simulink model "ex_9_3"  (Simulink 10.1)
settings: Solver=ode23  StartTime=0.0  StopTime=3  FixedStep=0.001  RelTol=1e-3
values from neighbouring files (symbols this model uses):
  a1 = I1 + m1 * Icl^2 + Ie + me * Ice^2 + me * L1^2    (= 3.34)    [ex_9_1.m]    (also in ex_9_2.m; ex_9_3.m)
  a2 = Ie + me * Ice^2    (= 0.97)    [ex_9_1.m]    (also in ex_9_2.m; ex_9_3.m)
  a3 = me * L1 * Ice * cos(delta_e)    [ex_9_1.m]    (also in ex_9_2.m = me_hat * L1 * Ice * cos(delta_e); ex_9_3.m = me_hat * L1 * Ice * cos(delta_e))
  a4 = me * L1 * Ice * sin(delta_e)    [ex_9_1.m]    (also in ex_9_2.m = me_hat * L1 * Ice * sin(delta_e); ex_9_3.m = me_hat * L1 * Ice * sin(delta_e))
  delta_e = 30    [ex_9_1.m]    (also in ex_9_2.m = 0.523599; ex_9_3.m = 0.523599)
  I1 = 0.12    [ex_9_1.m]    (also in ex_9_2.m; ex_9_3.m)
  Ice = 0.6    [ex_9_1.m]    (also in ex_9_2.m; ex_9_3.m)
  Icl = 0.5    [ex_9_1.m]    (also in ex_9_2.m; ex_9_3.m)
  Ie = 0.25    [ex_9_1.m]    (also in ex_9_2.m; ex_9_3.m)
  L1 = 1    [ex_9_1.m]    (also in ex_9_2.m; ex_9_3.m)
libraries: dspmtrx3 x4
settings Model: Creator=Paulo Padrao  LastModifiedBy=Paulo Padrao
settings DataIOCC: SaveFormat=Dataset
settings OptimizationCC: LifeSpan=auto
settings DebuggingCC: UnderspecifiedInitializationDetection=Simplified  MergeDetectMultiDrivingBlocksExec=error  SFUnexpectedBacktrackingDiag=error  SFNoUnconditionalDefaultTransitionDiag=error  SFExecutionAtInitializationDiag=warning
settings HardwareCC: ProdBitPerPointer=64  ProdBitPerSizeT=64  ProdBitPerPtrDiffT=64  ProdLargestAtomicFloat=Float  ProdIntDivRoundTo=Zero  ProdEndianess=LittleEndian  ProdWordSize=64  ProdHWDeviceType=Intel->x86-64 (Windows64)
settings ModelReferenceCC: PropagateSignalLabelsOutOfModel=on
settings CodeAppCC: StateflowObjectComments=off
settings GRTTargetCC: TargetLangStandard=C99 (ISO)  CombineOutputUpdateFcns=on  GRTInterface=off
settings ConfigComp: CovMetricSettings=dwe  CovHtmlReporting=off  CovSaveCumulativeToWorkspaceVar=off  CovSaveSingleToWorkspaceVar=off  CovExternalEMLEnable=on

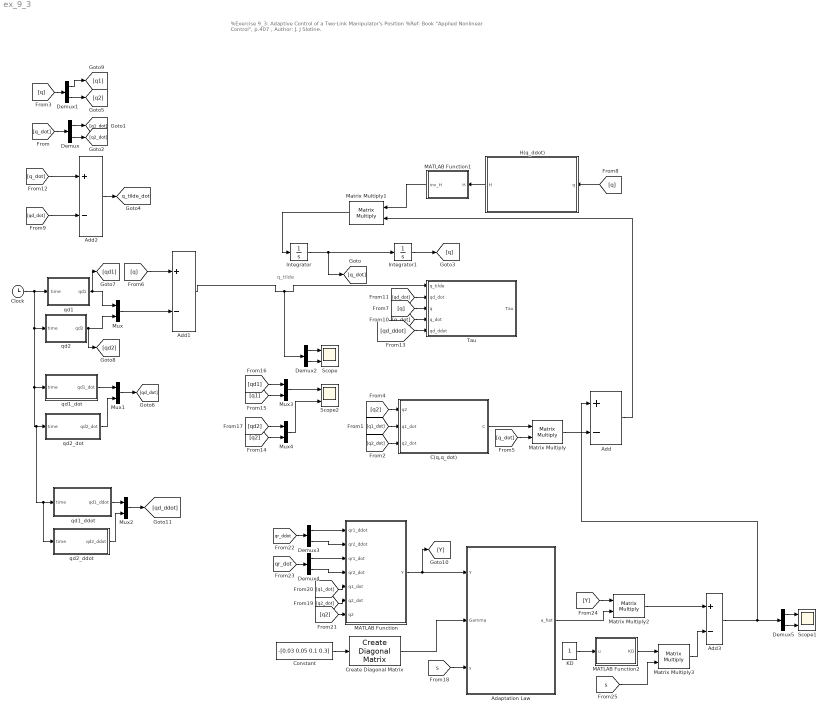
== system ex_9_3 ==
  note: %Exercise 9_3: Adaptive Control of a Two-Link Manipulator's Position
      | %Ref: Book "Applied Nonlinear Control", p.407 , Author: J. J Slotine.
  note: q_tilde
  Adaptation Law : Subsystem
  Add{,1..3} (4 alike) : Sum  Inputs=+-
  C(q,q_dot) : Subsystem
  Clock : Clock
  Constant : Constant  Value=-[0.03 0.05 0.1 0.3]
  Create Diagonal Matrix : dspmtrx3/Create Diagonal Matrix
      settings: SourceProductBaseCode=DS
  Demux{,1..5} (6 alike) : Demux  Outputs=2
  H(q_ddot) : Subsystem
  Integrator : Integrator
  Integrator1 : Integrator
  KD : Constant
  MATLAB Function : MATLAB Function  TreatAsAtomicUnit=on
  MATLAB Function1 : MATLAB Function  TreatAsAtomicUnit=on
  MATLAB Function2 : MATLAB Function  TreatAsAtomicUnit=on
  Matrix Multiply{,1..3} (4 alike) : Product  Multiplication=Matrix(*)
  Mux{,1..4} (5 alike) : Mux  Inputs=2
  Scope : Scope  NumInputPorts=2
  Scope1 : Scope  NumInputPorts=2
  Scope2 : Scope  NumInputPorts=2
  Tau : Subsystem
  qd1 : MATLAB Function  TreatAsAtomicUnit=on
  qd1_ddot : MATLAB Function  TreatAsAtomicUnit=on
  qd1_dot : MATLAB Function  TreatAsAtomicUnit=on
  qd2 : MATLAB Function  TreatAsAtomicUnit=on
  qd2_ddot : MATLAB Function  TreatAsAtomicUnit=on
  qd2_dot : MATLAB Function  TreatAsAtomicUnit=on
  tag scope: q_tilde_dot=global
  wires:
  Integrator/1 -> [q_dot], Integrator1/1
  [q_dot] -> Demux/1
  Demux/1 -> [q1_dot]
  Demux/2 -> [q2_dot]
  [q1_dot] -> C(q,q_dot)/2(q1_dot)
  [q2_dot] -> C(q,q_dot)/3(q2_dot)
  Integrator1/1 -> [q]
  [q] -> Demux1/1
  Demux1/2 -> [q2]
  [q2] -> C(q,q_dot)/1(q2)
  C(q,q_dot)/1(C) -> Matrix Multiply/1
  [q_dot] -> Matrix Multiply/2
  [q] -> H(q_ddot)/1(q)
  qd2/1(qd2) -> Mux/2, [qd2]
  [q] -> Add1/1
  Mux/1 -> Add1/2
  Add1/1 -> Demux2/1, Tau/1(q_tilde)
  [qd_dot] -> Tau/2(qd_dot)
  Demux1/1 -> [q1]
  Matrix Multiply/1 -> Add/2
  Matrix Multiply1/1 -> Integrator/1
  Add/1 -> Matrix Multiply1/2
  Demux2/2 -> Scope/2
  Demux2/1 -> Scope/1
  [q] -> Tau/3(q)
  [q_dot] -> Tau/4(q_dot)
  qd1_dot/1(qd1_dot) -> Mux1/1
  qd2_dot/1(qd2_dot) -> Mux1/2
  Mux1/1 -> [qd_dot]
  H(q_ddot)/1(H) -> MATLAB Function1/1(H)
  MATLAB Function1/1(inv_H) -> Matrix Multiply1/1
  [qd_dot] -> Add2/2
  [q_dot] -> Add2/1
  Add2/1 -> [q_tilde_dot]
  Clock/1 -> qd2_ddot/1(time), qd1_ddot/1(time), qd2_dot/1(time), qd1_dot/1(time), qd2/1(time), qd1/1(time)
  qd2_ddot/1(qd2_ddot) -> Mux2/2
  Mux2/1 -> [qd_ddot]
  qd1_ddot/1(qd1_ddot) -> Mux2/1
  [qd_ddot] -> Tau/5(qd_ddot)
  Mux3/1 -> Scope2/1
  qd1/1(qd1) -> Mux/1, [qd1]
  Mux4/1 -> Scope2/2
  [q2] -> Mux4/2
  [q1] -> Mux3/2
  [qd1] -> Mux3/1
  [qd2] -> Mux4/1
  Constant/1 -> Create Diagonal Matrix/1
  Create Diagonal Matrix/1 -> Adaptation Law/2(Gamma)
  [s] -> Adaptation Law/3(s)
  MATLAB Function/1(Y) -> [Y], Adaptation Law/1(Y)
  [q2_dot] -> MATLAB Function/6(q2_dot)
  [q1_dot] -> MATLAB Function/5(q1_dot)
  [q2] -> MATLAB Function/7(q2)
  [qr_ddot] -> Demux3/1
  Demux3/1 -> MATLAB Function/1(qr1_ddot)
  Demux3/2 -> MATLAB Function/2(qr2_ddot)
  Demux4/2 -> MATLAB Function/4(qr2_dot)
  Demux4/1 -> MATLAB Function/3(qr1_dot)
  [qr_dot] -> Demux4/1
  [Y] -> Matrix Multiply2/1
  Adaptation Law/1(a_hat) -> Matrix Multiply2/2
  Matrix Multiply2/1 -> Add3/1
  Demux5/1 -> Scope1/1
  Demux5/2 -> Scope1/2
  Add3/1 -> Add/1, Demux5/1
  Matrix Multiply3/1 -> Add3/2
  MATLAB Function2/1(KD) -> Matrix Multiply3/1
  [s] -> Matrix Multiply3/2
  KD/1 -> MATLAB Function2/1(u)

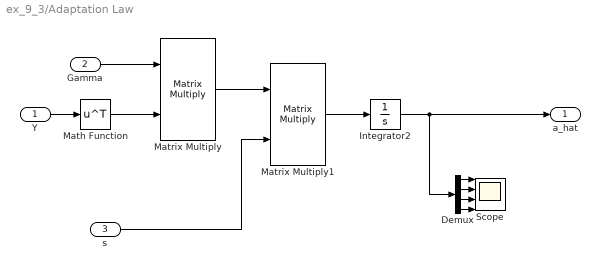
== system ex_9_3/Adaptation Law ==
  Y : Inport
  Gamma : Inport  Port=2
  s : Inport  Port=3
  Demux : Demux
  Integrator2 : Integrator
  Math Function : Math  Operator=transpose  SignedPower=on  SaturateOnIntegerOverflow=on
  Matrix Multiply : Product  Multiplication=Matrix(*)
  Matrix Multiply1 : Product  Multiplication=Matrix(*)
  Scope : Scope  NumInputPorts=4
  a_hat : Outport  VectorParamsAs1DForOutWhenUnconnected=off
  wires:
  Integrator2/1 -> Demux/1, a_hat/1
  Gamma/1 -> Matrix Multiply/1
  Math Function/1 -> Matrix Multiply/2
  Y/1 -> Math Function/1
  Matrix Multiply/1 -> Matrix Multiply1/1
  s/1 -> Matrix Multiply1/2
  Matrix Multiply1/1 -> Integrator2/1
  Demux/1 -> Scope/1
  Demux/2 -> Scope/2
  Demux/3 -> Scope/3
  Demux/4 -> Scope/4

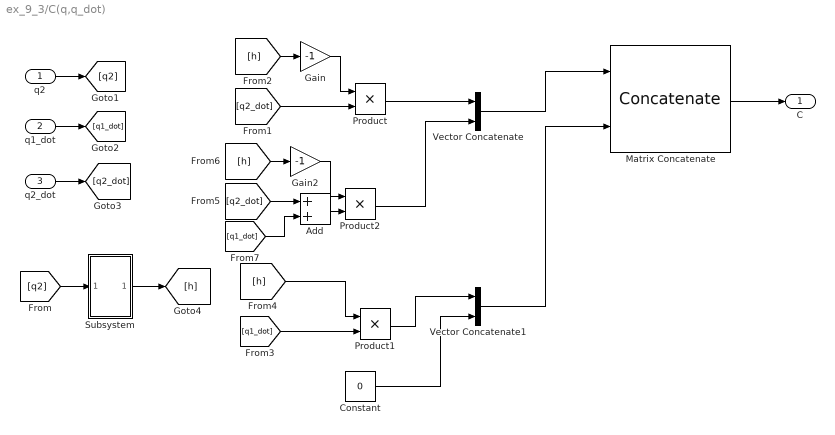
== system ex_9_3/C(q,q_dot) ==
  q2 : Inport
  q1_dot : Inport  Port=2
  q2_dot : Inport  Port=3
  Add : Sum
  Constant : Constant  Value=0
  Gain : Gain  Gain=-1
  Gain2 : Gain  Gain=-1
  Matrix Concatenate : Concatenate  Mode=Multidimensional array
  Product : Product
  Product1 : Product
  Product2 : Product
  Subsystem : Subsystem
  Vector Concatenate : Concatenate  Mode=Multidimensional array  ConcatenateDimension=2
  Vector Concatenate1 : Concatenate  Mode=Multidimensional array  ConcatenateDimension=2
  C : Outport  VectorParamsAs1DForOutWhenUnconnected=off
  wires:
  q2/1 -> [q2]
  q1_dot/1 -> [q1_dot]
  q2_dot/1 -> [q2_dot]
  [q2] -> Subsystem/1(In1)
  Subsystem/1(Out1) -> [h]
  Matrix Concatenate/1 -> C/1
  [q2_dot] -> Product/2
  [h] -> Gain/1
  Gain/1 -> Product/1
  [h] -> Product1/1
  [q1_dot] -> Product1/2
  Gain2/1 -> Product2/1
  [h] -> Gain2/1
  [q2_dot] -> Add/1
  [q1_dot] -> Add/2
  Add/1 -> Product2/2
  Product/1 -> Vector Concatenate/1
  Vector Concatenate/1 -> Matrix Concatenate/1
  Constant/1 -> Vector Concatenate1/2
  Vector Concatenate1/1 -> Matrix Concatenate/2
  Product2/1 -> Vector Concatenate/2
  Product1/1 -> Vector Concatenate1/1

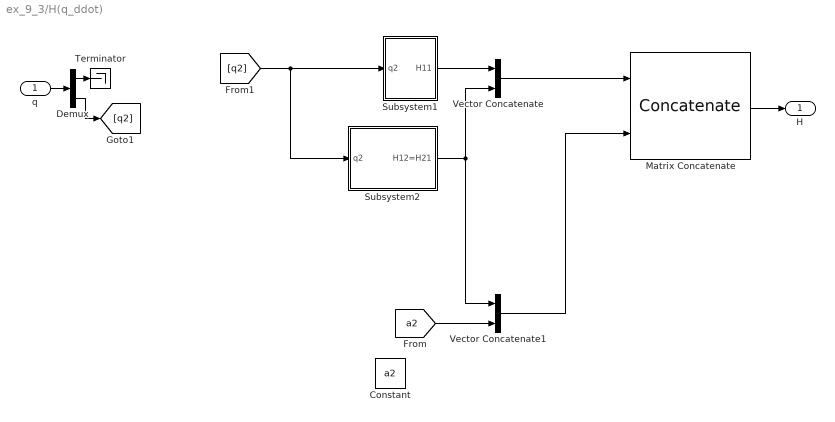
== system ex_9_3/H(q_ddot) ==
  q : Inport
  Constant : Constant  Value=a2
  Demux : Demux  Outputs=2
  Matrix Concatenate : Concatenate  Mode=Multidimensional array
  Subsystem1 : Subsystem
  Subsystem2 : Subsystem
  Terminator : Terminator
  Vector Concatenate : Concatenate  Mode=Multidimensional array  ConcatenateDimension=2
  Vector Concatenate1 : Concatenate  Mode=Multidimensional array  ConcatenateDimension=2
  H : Outport  VectorParamsAs1DForOutWhenUnconnected=off
  wires:
  q/1 -> Demux/1
  Demux/2 -> [q2]
  [q2] -> Subsystem1/1(q2), Subsystem2/1(q2)
  Subsystem2/1("H12=H21 ") -> Vector Concatenate1/1, Vector Concatenate/2
  Vector Concatenate1/1 -> Matrix Concatenate/2
  Subsystem1/1("H11 ") -> Vector Concatenate/1
  Vector Concatenate/1 -> Matrix Concatenate/1
  Demux/1 -> Terminator/1
  Matrix Concatenate/1 -> H/1
  [a2] -> Vector Concatenate1/2

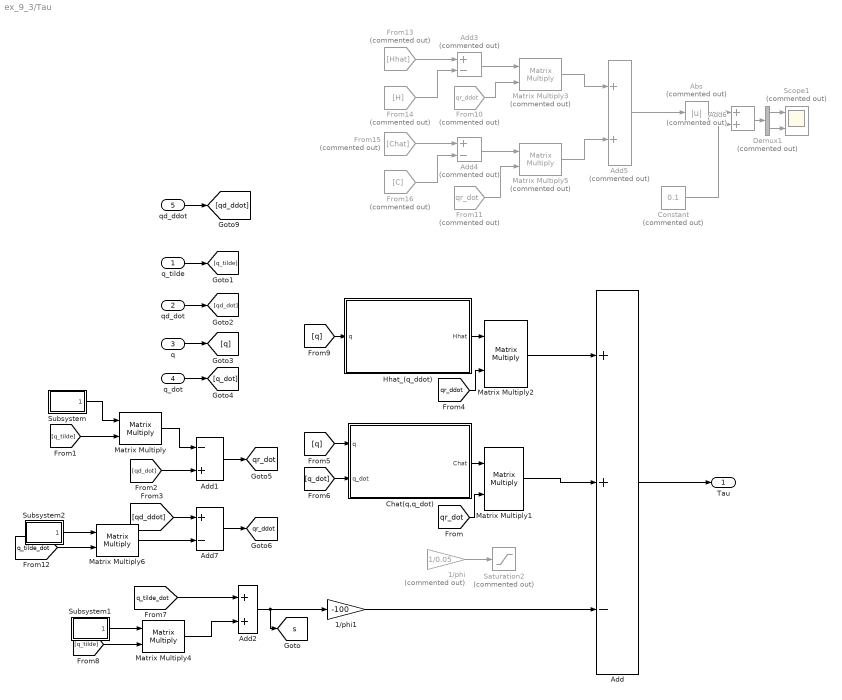
== system ex_9_3/Tau ==
  q_tilde : Inport
  qd_dot : Inport  Port=2
  q : Inport  Port=3
  q_dot : Inport  Port=4
  qd_ddot : Inport  Port=5
  1/phi : Gain  Commented=on  Gain=1/0.05
  1/phi1 : Gain  Gain=-100
  Abs : Abs  Commented=on  ZeroCross=off
  Add : Sum  Inputs=++-
  Add1 : Sum  Inputs=-+
  Add2 : Sum
  Add3 : Sum  Commented=on  Inputs=+-
  Add4 : Sum  Commented=on  Inputs=+-
  Add5 : Sum  Commented=on
  Add6 : Sum  Commented=on
  Add7 : Sum  Inputs=+-
  Chat(q,q_dot) : Subsystem
  Constant : Constant  Commented=on  Value=0.1
  Demux1 : Demux  Commented=on  Outputs=2
  From10 : From  Commented=on  GotoTag=qr_ddot
  From11 : From  Commented=on  GotoTag=qr_dot
  From13 : From  Commented=on  GotoTag=Hhat  TagVisibility=global
  From14 : From  Commented=on  GotoTag=H  TagVisibility=global
  From15 : From  Commented=on  GotoTag=Chat  TagVisibility=global
  From16 : From  Commented=on  GotoTag=C  TagVisibility=global
  Hhat_(q_ddot) : Subsystem
  Matrix Multiply{,1..2,4,6} (5 alike) : Product  Multiplication=Matrix(*)
  Matrix Multiply3 : Product  Commented=on  Multiplication=Matrix(*)
  Matrix Multiply5 : Product  Commented=on  Multiplication=Matrix(*)
  Saturation2 : Saturate  Commented=on  UpperLimit=0.1  LowerLimit=-0.1  LinearizeAsGain=off  ZeroCross=off
  Scope1 : Scope  Commented=on  NumInputPorts=2
  Subsystem : Subsystem
  Subsystem1 : Subsystem
  Subsystem2 : Subsystem
  Tau : Outport  VectorParamsAs1DForOutWhenUnconnected=off
  tag scope: qr_ddot=global, qr_dot=global, s=global
  wires:
  Add/1 -> Tau/1
  q_tilde/1 -> [q_tilde]
  qd_dot/1 -> [qd_dot]
  [q_tilde] -> Matrix Multiply/2
  q/1 -> [q]
  q_dot/1 -> [q_dot]
  Subsystem/1(lambda) -> Matrix Multiply/1
  Matrix Multiply/1 -> Add1/1
  Add1/1 -> [qr_dot]
  Matrix Multiply2/1 -> Add/1
  Matrix Multiply1/1 -> Add/2
  [qr_dot] -> Matrix Multiply1/2
  [qr_ddot] -> Matrix Multiply2/2
  Chat(q,q_dot)/1(Chat) -> Matrix Multiply1/1
  [q] -> Chat(q,q_dot)/1(q)
  [q_dot] -> Chat(q,q_dot)/2(q_dot)
  [q_tilde_dot] -> Add2/1
  Matrix Multiply4/1 -> Add2/2
  Hhat_(q_ddot)/1(Hhat) -> Matrix Multiply2/1
  [q] -> Hhat_(q_ddot)/1(q)
  [qd_dot] -> Add1/2
  Subsystem1/1(lambda) -> Matrix Multiply4/1
  [q_tilde] -> Matrix Multiply4/2
  1/phi/1 -> Saturation2/1
  From13/1 -> Add3/1
  From16/1 -> Add4/2
  From15/1 -> Add4/1
  Add3/1 -> Matrix Multiply3/1
  From14/1 -> Add3/2
  From10/1 -> Matrix Multiply3/2
  Add4/1 -> Matrix Multiply5/1
  From11/1 -> Matrix Multiply5/2
  Matrix Multiply3/1 -> Add5/1
  Matrix Multiply5/1 -> Add5/2
  Add5/1 -> Abs/1
  Abs/1 -> Add6/1
  Constant/1 -> Add6/2
  qd_ddot/1 -> [qd_ddot]
  Add7/1 -> [qr_ddot]
  [qd_ddot] -> Add7/1
  Matrix Multiply6/1 -> Add7/2
  Subsystem2/1(lambda) -> Matrix Multiply6/1
  [q_tilde_dot] -> Matrix Multiply6/2
  Add6/1 -> Demux1/1
  Demux1/1 -> Scope1/1
  Demux1/2 -> Scope1/2
  1/phi1/1 -> Add/3
  Add2/1 -> [s], 1/phi1/1

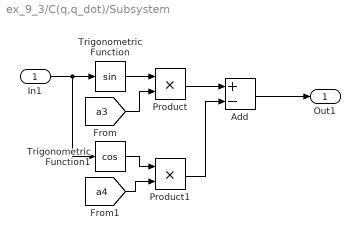
== system ex_9_3/C(q,q_dot)/Subsystem ==
  In1 : Inport
  Add : Sum  Inputs=+-
  Product : Product
  Product1 : Product
  Trigonometric Function : Trigonometry
  Trigonometric Function1 : Trigonometry  Operator=cos
  Out1 : Outport  VectorParamsAs1DForOutWhenUnconnected=off
  wires:
  Trigonometric Function1/1 -> Product1/1
  [a3] -> Product/2
  Product/1 -> Add/1
  [a4] -> Product1/2
  In1/1 -> Trigonometric Function1/1, Trigonometric Function/1
  Trigonometric Function/1 -> Product/1
  Add/1 -> Out1/1
  Product1/1 -> Add/2

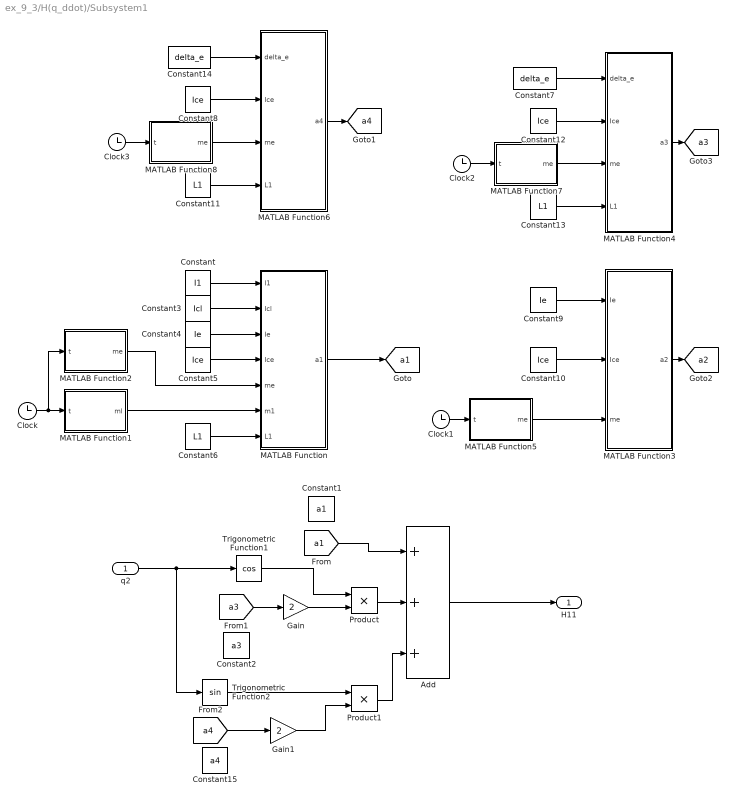
== system ex_9_3/H(q_ddot)/Subsystem1 ==
  q2 : Inport
  Add : Sum  Inputs=+++
  Clock{,1..3} (4 alike) : Clock
  Constant : Constant  Value=I1
  Constant1 : Constant  Value=a1
  Constant{5,8,10,12} (4 alike) : Constant  Value=Ice
  Constant11 : Constant  Value=L1
  Constant13 : Constant  Value=L1
  Constant14 : Constant  Value=delta_e
  Constant15 : Constant  Value=a4
  Constant2 : Constant  Value=a3
  Constant3 : Constant  Value=Icl
  Constant4 : Constant  Value=Ie
  Constant6 : Constant  Value=L1
  Constant7 : Constant  Value=delta_e
  Constant9 : Constant  Value=Ie
  Gain : Gain  Gain=2
  Gain1 : Gain  Gain=2
  MATLAB Function : MATLAB Function  TreatAsAtomicUnit=on
  MATLAB Function1 : MATLAB Function  TreatAsAtomicUnit=on
  MATLAB Function2 : MATLAB Function  TreatAsAtomicUnit=on
  MATLAB Function3 : MATLAB Function  TreatAsAtomicUnit=on
  MATLAB Function4 : MATLAB Function  TreatAsAtomicUnit=on
  MATLAB Function5 : MATLAB Function  TreatAsAtomicUnit=on
  MATLAB Function6 : MATLAB Function  TreatAsAtomicUnit=on
  MATLAB Function7 : MATLAB Function  TreatAsAtomicUnit=on
  MATLAB Function8 : MATLAB Function  TreatAsAtomicUnit=on
  Product : Product
  Product1 : Product
  Trigonometric Function1 : Trigonometry  Operator=cos
  Trigonometric Function2 : Trigonometry
  "H11 " : Outport  VectorParamsAs1DForOutWhenUnconnected=off
  tag scope: a1=global, a2=global, a3=global, a4=global
  wires:
  q2/1 -> Trigonometric Function1/1, Trigonometric Function2/1
  Add/1 -> "H11 "/1
  Product/1 -> Add/2
  Trigonometric Function1/1 -> Product/1
  Trigonometric Function2/1 -> Product1/1
  Product1/1 -> Add/3
  Constant/1 -> MATLAB Function/1(I1)
  Constant3/1 -> MATLAB Function/2(Icl)
  Constant4/1 -> MATLAB Function/3(Ie)
  Constant5/1 -> MATLAB Function/4(Ice)
  Constant6/1 -> MATLAB Function/7(L1)
  Clock/1 -> MATLAB Function2/1(t), MATLAB Function1/1(t)
  MATLAB Function1/1(ml) -> MATLAB Function/6(m1)
  MATLAB Function2/1(me) -> MATLAB Function/5(me)
  MATLAB Function5/1(me) -> MATLAB Function3/3(me)
  Clock1/1 -> MATLAB Function5/1(t)
  Constant10/1 -> MATLAB Function3/2(Ice)
  Constant9/1 -> MATLAB Function3/1(Ie)
  MATLAB Function7/1(me) -> MATLAB Function4/3(me)
  Clock2/1 -> MATLAB Function7/1(t)
  Constant13/1 -> MATLAB Function4/4(L1)
  Constant12/1 -> MATLAB Function4/2(Ice)
  Constant7/1 -> MATLAB Function4/1(delta_e)
  Constant14/1 -> MATLAB Function6/1(delta_e)
  Constant8/1 -> MATLAB Function6/2(Ice)
  Constant11/1 -> MATLAB Function6/4(L1)
  Clock3/1 -> MATLAB Function8/1(t)
  MATLAB Function8/1(me) -> MATLAB Function6/3(me)
  MATLAB Function/1(a1) -> [a1]
  MATLAB Function6/1(a4) -> [a4]
  MATLAB Function3/1(a2) -> [a2]
  MATLAB Function4/1(a3) -> [a3]
  Gain/1 -> Product/2
  Gain1/1 -> Product1/2
  [a4] -> Gain1/1
  [a3] -> Gain/1
  [a1] -> Add/1

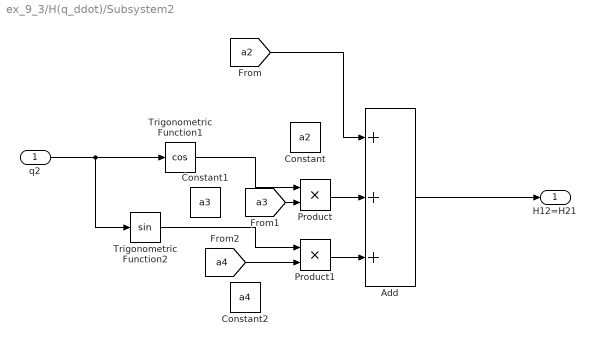
== system ex_9_3/H(q_ddot)/Subsystem2 ==
  q2 : Inport
  Add : Sum  Inputs=+++
  Constant : Constant  Value=a2
  Constant1 : Constant  Value=a3
  Constant2 : Constant  Value=a4
  Product : Product
  Product1 : Product
  Trigonometric Function1 : Trigonometry  Operator=cos
  Trigonometric Function2 : Trigonometry
  "H12=H21 " : Outport  VectorParamsAs1DForOutWhenUnconnected=off
  wires:
  Product1/1 -> Add/3
  Trigonometric Function2/1 -> Product1/1
  Trigonometric Function1/1 -> Product/1
  Product/1 -> Add/2
  Add/1 -> "H12=H21 "/1
  q2/1 -> Trigonometric Function2/1, Trigonometric Function1/1
  [a4] -> Product1/2
  [a3] -> Product/2
  [a2] -> Add/1

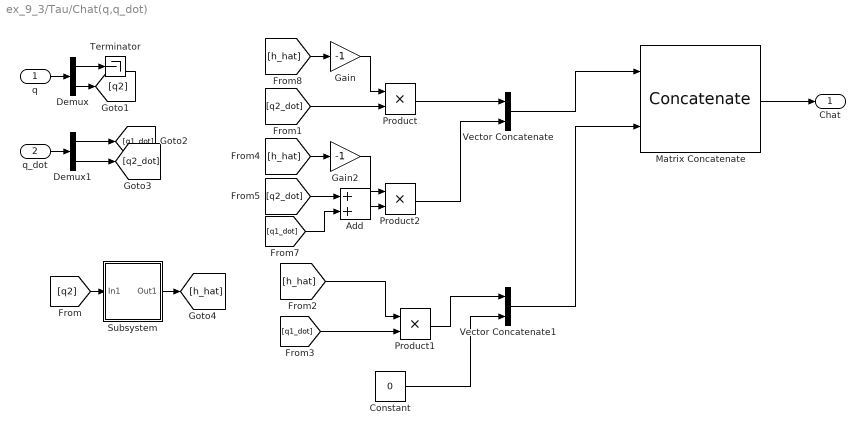
== system ex_9_3/Tau/Chat(q,q_dot) ==
  q : Inport
  q_dot : Inport  Port=2
  Add : Sum
  Constant : Constant  Value=0
  Demux : Demux  Outputs=2
  Demux1 : Demux  Outputs=2
  Gain : Gain  Gain=-1
  Gain2 : Gain  Gain=-1
  Matrix Concatenate : Concatenate  Mode=Multidimensional array
  Product : Product
  Product1 : Product
  Product2 : Product
  Subsystem : Subsystem
  Terminator : Terminator
  Vector Concatenate : Concatenate  Mode=Multidimensional array  ConcatenateDimension=2
  Vector Concatenate1 : Concatenate  Mode=Multidimensional array  ConcatenateDimension=2
  Chat : Outport  VectorParamsAs1DForOutWhenUnconnected=off
  wires:
  [q2] -> Subsystem/1(In1)
  Subsystem/1(Out1) -> [h_hat]
  Matrix Concatenate/1 -> Chat/1
  [q2_dot] -> Product/2
  [h_hat] -> Gain/1
  Gain/1 -> Product/1
  [h_hat] -> Product1/1
  [q1_dot] -> Product1/2
  Gain2/1 -> Product2/1
  [h_hat] -> Gain2/1
  [q2_dot] -> Add/1
  [q1_dot] -> Add/2
  Add/1 -> Product2/2
  Product/1 -> Vector Concatenate/1
  Vector Concatenate/1 -> Matrix Concatenate/1
  Constant/1 -> Vector Concatenate1/2
  Vector Concatenate1/1 -> Matrix Concatenate/2
  q/1 -> Demux/1
  Demux/2 -> [q2]
  Demux/1 -> Terminator/1
  q_dot/1 -> Demux1/1
  Demux1/2 -> [q2_dot]
  Demux1/1 -> [q1_dot]
  Product1/1 -> Vector Concatenate1/1
  Product2/1 -> Vector Concatenate/2

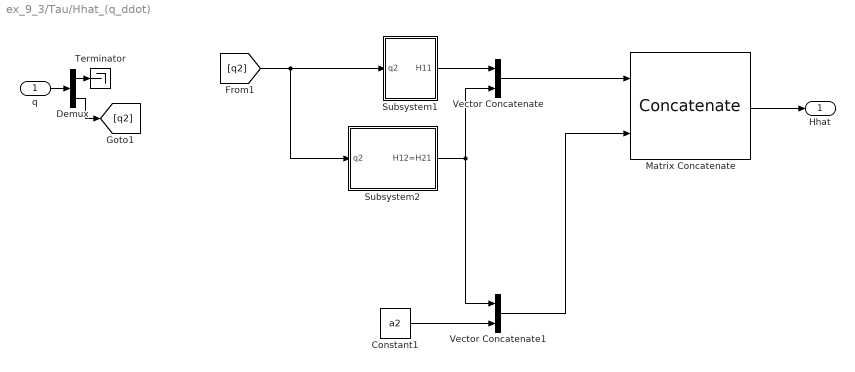
== system ex_9_3/Tau/Hhat_(q_ddot) ==
  q : Inport
  Constant1 : Constant  Value=a2
  Demux : Demux  Outputs=2
  Matrix Concatenate : Concatenate  Mode=Multidimensional array
  Subsystem1 : Subsystem
  Subsystem2 : Subsystem
  Terminator : Terminator
  Vector Concatenate : Concatenate  Mode=Multidimensional array  ConcatenateDimension=2
  Vector Concatenate1 : Concatenate  Mode=Multidimensional array  ConcatenateDimension=2
  Hhat : Outport  VectorParamsAs1DForOutWhenUnconnected=off
  wires:
  Vector Concatenate1/1 -> Matrix Concatenate/2
  Vector Concatenate/1 -> Matrix Concatenate/1
  Matrix Concatenate/1 -> Hhat/1
  Subsystem1/1("H11 ") -> Vector Concatenate/1
  [q2] -> Subsystem1/1(q2), Subsystem2/1(q2)
  Constant1/1 -> Vector Concatenate1/2
  Subsystem2/1("H12=H21 ") -> Vector Concatenate1/1, Vector Concatenate/2
  q/1 -> Demux/1
  Demux/2 -> [q2]
  Demux/1 -> Terminator/1

== system ex_9_3/Tau/Subsystem ==
  Identity Matrix2 : dspmtrx3/Identity Matrix  Inherit=off  N=2  Ts=1  dataType=double  isSigned=on  wordLen=16  udDataType=sfix(16)  fracBitsMode=Best precision  numFracBits=15  OutDataTypeStr=double  LastOutDataTypeStr=double
  LAMBDA : Constant  Value=20
  Product1 : Product
  lambda : Outport  VectorParamsAs1DForOutWhenUnconnected=off
  wires:
  Identity Matrix2/1 -> Product1/1
  LAMBDA/1 -> Product1/2
  Product1/1 -> lambda/1

== system ex_9_3/Tau/Subsystem1 ==
  Identity Matrix2 : dspmtrx3/Identity Matrix  Inherit=off  N=2  Ts=1  dataType=double  isSigned=on  wordLen=16  udDataType=sfix(16)  fracBitsMode=Best precision  numFracBits=15  OutDataTypeStr=double  LastOutDataTypeStr=double
  LAMBDA : Constant  Value=20
  Product1 : Product
  lambda : Outport  VectorParamsAs1DForOutWhenUnconnected=off
  wires:
  Product1/1 -> lambda/1
  LAMBDA/1 -> Product1/2
  Identity Matrix2/1 -> Product1/1

== system ex_9_3/Tau/Subsystem2 ==
  Identity Matrix2 : dspmtrx3/Identity Matrix  Inherit=off  N=2  Ts=1  dataType=double  isSigned=on  wordLen=16  udDataType=sfix(16)  fracBitsMode=Best precision  numFracBits=15  OutDataTypeStr=double  LastOutDataTypeStr=double
  LAMBDA : Constant  Value=20
  Product1 : Product
  lambda : Outport  VectorParamsAs1DForOutWhenUnconnected=off
  wires:
  Product1/1 -> lambda/1
  LAMBDA/1 -> Product1/2
  Identity Matrix2/1 -> Product1/1

== system ex_9_3/Tau/Chat(q,q_dot)/Subsystem ==
  In1 : Inport
  Add : Sum  Inputs=+-
  Constant : Constant  Value=a3
  Constant1 : Constant  Value=a4
  Product : Product
  Product1 : Product
  Trigonometric Function : Trigonometry
  Trigonometric Function1 : Trigonometry  Operator=cos
  Out1 : Outport  VectorParamsAs1DForOutWhenUnconnected=off
  wires:
  Trigonometric Function1/1 -> Product1/1
  Constant/1 -> Product/2
  Product/1 -> Add/1
  Constant1/1 -> Product1/2
  In1/1 -> Trigonometric Function1/1, Trigonometric Function/1
  Trigonometric Function/1 -> Product/1
  Add/1 -> Out1/1
  Product1/1 -> Add/2

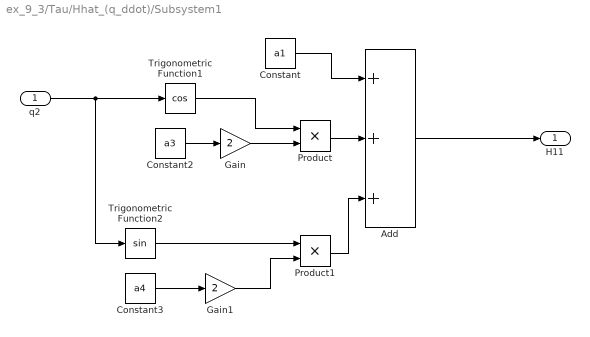
== system ex_9_3/Tau/Hhat_(q_ddot)/Subsystem1 ==
  q2 : Inport
  Add : Sum  Inputs=+++
  Constant : Constant  Value=a1
  Constant2 : Constant  Value=a3
  Constant3 : Constant  Value=a4
  Gain : Gain  Gain=2
  Gain1 : Gain  Gain=2
  Product : Product
  Product1 : Product
  Trigonometric Function1 : Trigonometry  Operator=cos
  Trigonometric Function2 : Trigonometry
  "H11 " : Outport  VectorParamsAs1DForOutWhenUnconnected=off
  wires:
  q2/1 -> Trigonometric Function1/1, Trigonometric Function2/1
  Add/1 -> "H11 "/1
  Product/1 -> Add/2
  Trigonometric Function1/1 -> Product/1
  Constant2/1 -> Gain/1
  Constant3/1 -> Gain1/1
  Trigonometric Function2/1 -> Product1/1
  Product1/1 -> Add/3
  Constant/1 -> Add/1
  Gain/1 -> Product/2
  Gain1/1 -> Product1/2

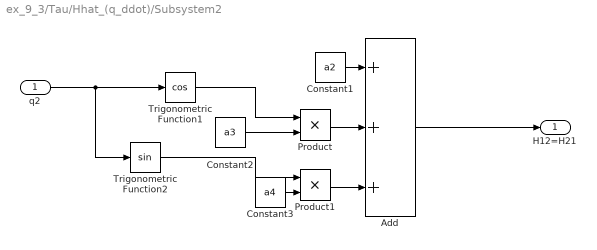
== system ex_9_3/Tau/Hhat_(q_ddot)/Subsystem2 ==
  q2 : Inport
  Add : Sum  Inputs=+++
  Constant1 : Constant  Value=a2
  Constant2 : Constant  Value=a3
  Constant3 : Constant  Value=a4
  Product : Product
  Product1 : Product
  Trigonometric Function1 : Trigonometry  Operator=cos
  Trigonometric Function2 : Trigonometry
  "H12=H21 " : Outport  VectorParamsAs1DForOutWhenUnconnected=off
  wires:
  Product1/1 -> Add/3
  Trigonometric Function2/1 -> Product1/1
  Constant2/1 -> Product/2
  Trigonometric Function1/1 -> Product/1
  Product/1 -> Add/2
  Add/1 -> "H12=H21 "/1
  q2/1 -> Trigonometric Function2/1, Trigonometric Function1/1
  Constant1/1 -> Add/1
  Constant3/1 -> Product1/2

== matlab function qd1 ==
  data: time input double; qd1 output double
function qd1 = fcn(time)

qd1 = 30*(1-cos(2*pi*time));

== matlab function MATLAB Function ==
  data: qr1_ddot input double; Y output double; qr2_ddot input double; qr1_dot input double; qr2_dot input double; q1_dot input double; q2_dot input double; q2 input double
function Y = fcn(qr1_ddot, qr2_ddot, qr1_dot,qr2_dot,q1_dot,q2_dot,q2)


Y11 = qr1_ddot;
Y12 = qr2_ddot;
Y13 = (2*qr1_ddot + qr2_ddot)*cos(q2) ...
    - (q2_dot*qr1_dot + q1_dot*qr2_dot + q2_dot*qr2_dot)*sin(q2);

Y14 = (2*qr1_ddot + qr2_ddot)*sin(q2) ...
    + (q2_dot*qr1_dot + q1_dot*qr2_dot + q2_dot*qr2_dot)*cos(q2);

Y21 = 0;
Y22 = qr1_ddot + qr2_ddot;
Y23 = qr1_ddot*cos(q2) + q1_dot*qr1_dot*sin(q2);
Y24 = qr1_ddot*sin(q2) - q1_dot*qr1_dot*cos(q2);

Y = [Y11 Y12 Y13 Y14;
     Y21 Y22 Y23 Y24];

== matlab function qd2 ==
  data: time input double; qd2 output double
function qd2 = fcn(time)

qd2 = 45*(1-cos(2*pi*time));

== matlab function qd2_dot ==
  data: time input double; qd2_dot output double
function qd2_dot = fcn(time)

qd2_dot = 90*pi*sin(2*pi*time);

== matlab function qd1_dot ==
  data: time input double; qd1_dot output double
function qd1_dot = fcn(time)

qd1_dot = 60*pi*sin(2*pi*time);

== matlab function MATLAB Function1 ==
  data: H input double; inv_H output double size=2,2
function inv_H = inv(H)

inv_H = inv(H);

== matlab function MATLAB Function2 ==
  data: u input double; KD output double
function KD = fcn(u)

KD = u*eye(2);

== matlab function qd1_ddot ==
  data: time input double; qd1_ddot output double
function qd1_ddot = fcn(time)

qd1_ddot = 120*pi^2*cos(2*pi*time);

== matlab function qd2_ddot ==
  data: time input double; qd2_ddot output double
function qd2_ddot = fcn(time)

qd2_ddot = 180*pi^2*cos(2*pi*time);

== matlab function H(q_ddot)/Subsystem1/MATLAB Function ==
  data: I1 input double; a1 output double; Icl input double; Ie input double; Ice input double; me input double; m1 input double; L1 input double
function a1 = fcn(I1,Icl,Ie,Ice,me,m1,L1)



a1 = I1 + m1*Icl^2 + Ie + me*Ice^2 + me*L1^2;

== matlab function H(q_ddot)/Subsystem1/MATLAB Function1 ==
  data: t input double; ml output double
function ml = fcn(t)

ml = abs(sin(t)/2) + 0.8;

== matlab function H(q_ddot)/Subsystem1/MATLAB Function2 ==
  data: t input double; me output double
function me = fcn(t)

me = abs(sin(t)) + 1.6;

== matlab function H(q_ddot)/Subsystem1/MATLAB Function3 ==
  data: a2 output double; Ie input double; Ice input double; me input double
function a2 = fcn(Ie,Ice,me)



a2 = Ie +me*Ice^2;

== matlab function H(q_ddot)/Subsystem1/MATLAB Function4 ==
  data: delta_e input double; a3 output double; Ice input double; me input double; L1 input double
function a3 = fcn(delta_e,Ice,me,L1)



a3 = me*L1*Ice*cos(delta_e);

== matlab function H(q_ddot)/Subsystem1/MATLAB Function5 ==
  data: t input double; me output double
function me = fcn(t)

me = abs(sin(t)) + 1.6;

== matlab function H(q_ddot)/Subsystem1/MATLAB Function6 ==
  data: delta_e input double; a4 output double; Ice input double; me input double; L1 input double
function a4 = fcn(delta_e,Ice,me,L1)



a4 = me*L1*Ice*sin(delta_e);

== matlab function H(q_ddot)/Subsystem1/MATLAB Function7 ==
  data: t input double; me output double
function me = fcn(t)

me = abs(sin(t)) + 1.6;

== matlab function H(q_ddot)/Subsystem1/MATLAB Function8 ==
  data: t input double; me output double
function me = fcn(t)

me = abs(sin(t)) + 1.6;
